simulink model "OR_6s_30l"  (R2023b)
settings: Solver=VariableStepAuto  StartTime=0.0  StopTime=10.0  RelTol=1e-3
libraries: ABB_UPPAAL_Library x76
(part 2 of 2)

== matlab function OR_6s_30l/Bus_1 ==
  data: u input; y output
function y = fcn(u)

y = u;

== matlab function OR_6s_30l/Bus_14 ==
  data: u input; y output
function y = fcn(u)

y = u;

== matlab function OR_6s_30l/Bus_15 ==
  data: u input; y output
function y = fcn(u)

y = u;

== matlab function OR_6s_30l/Bus_16 ==
  data: u input; y output
function y = fcn(u)

y = u;

== matlab function OR_6s_30l/Bus_17 ==
  data: data input; u input; y output
function y = fcn(data, u)

y = u;

== matlab function OR_6s_30l/Bus_18 ==
  data: u input; y output
function y = fcn(u)

y = u;

== matlab function OR_6s_30l/Bus_19 ==
  data: u input; y output
function y = fcn(u)

y = u;

== matlab function OR_6s_30l/Bus_20 ==
  data: u input; y output
function y = fcn(u)

y = u;

== matlab function OR_6s_30l/Bus_21 ==
  data: u input; y output
function y = fcn(u)

y = u;

== matlab function OR_6s_30l/Bus_22 ==
  data: u input; y output
function y = fcn(u)

y = u;

== matlab function OR_6s_30l/Bus_23 ==
  data: u input; y output
function y = fcn(u)

y = u;

== matlab function OR_6s_30l/Bus_2 ==
  data: u input; y output
function y = fcn(u)

y = u;

== matlab function OR_6s_30l/Bus_24 ==
  data: data input; u input; y output
function y = fcn(data, u)

y = u;

== matlab function OR_6s_30l/Bus_25 ==
  data: data input; u input; y output
function y = fcn(data, u)

y = u;

== matlab function OR_6s_30l/Bus_26 ==
  data: u input; y output
function y = fcn(u)

y = u;

== matlab function OR_6s_30l/Bus_27 ==
  data: u input; y output
function y = fcn(u)

y = u;

== matlab function OR_6s_30l/Bus_28 ==
  data: u input; y output
function y = fcn(u)

y = u;

== matlab function OR_6s_30l/Bus_29 ==
  data: u input; y output
function y = fcn(u)

y = u;

== matlab function OR_6s_30l/Bus_30 ==
  data: u input; y output
function y = fcn(u)

y = u;

== matlab function OR_6s_30l/Bus_3 ==
  data: u input; y output
function y = fcn(u)

y = u;

== matlab function OR_6s_30l/Bus_4 ==
  data: data input; u input; y output
function y = fcn(data, u)

y = u;

== matlab function OR_6s_30l/Bus_5 ==
  data: u input; y output
function y = fcn(u)

y = u;

== matlab function OR_6s_30l/Bus_6 ==
  data: u input; y output
function y = fcn(u)

y = u;

== matlab function OR_6s_30l/Bus_7 ==
  data: u input; y output
function y = fcn(u)

y = u;

== matlab function OR_6s_30l/Bus_8 ==
  data: u input; y output
function y = fcn(u)

y = u;

== matlab function OR_6s_30l/Bus_10 ==
  data: data input; u input; y output
function y = fcn(data, u)

y = u;

== matlab function OR_6s_30l/Bus_9 ==
  data: u input; y output
function y = fcn(u)

y = u;

== matlab function OR_6s_30l/Bus_11 ==
  data: u input; y output
function y = fcn(u)

y = u;

== matlab function OR_6s_30l/Bus_12 ==
  data: u input; y output
function y = fcn(u)

y = u;

== matlab function OR_6s_30l/Bus_13 ==
  data: u input; y output
function y = fcn(u)

y = u;
